simulink model "SistemaEstanques_PID_discreto"  (R2022a)
settings: Solver=ode3  StartTime=0.0  StopTime=3600*30  FixedStep=0.05  RelTol=1e-3  EnableMultiTasking=on
undefined symbols (not defined in the file or in its folder): gaussian, magnitude
libraries: simulink x5, slpidlib x1
settings Model: PauseTimes=10  PacingRate=100  Creator=Cristian  LastModifiedBy=Joaquín
settings SolverCC: AlgebraicLoopSolver=TrustRegion
settings DataIOCC: LimitDataPoints=on  SaveFormat=Array  ReturnWorkspaceOutputs=off
settings OptimizationCC: LifeSpan=inf
settings DebuggingCC: UnderspecifiedInitializationDetection=Classic  MergeDetectMultiDrivingBlocksExec=none  SolverPrmCheckMsg=warning  MultiTaskRateTransMsg=warning  UnconnectedInputMsg=warning  UnconnectedOutputMsg=warning  UnconnectedLineMsg=warning  StateNameClashWarn=warning  SFUnexpectedBacktrackingDiag=warning  SFNoUnconditionalDefaultTransitionDiag=warning  SFExecutionAtInitializationDiag=none  SFMachineParentedDataDiag=warning  ArithmeticOperatorsInVariantConditions=warning
settings HardwareCC: ProdBitPerPointer=32  ProdBitPerSizeT=32  ProdBitPerPtrDiffT=32  ProdLargestAtomicFloat=None  ProdIntDivRoundTo=Undefined  ProdEndianess=Unspecified  ProdWordSize=32  ProdHWDeviceType=32-bit Generic
settings ModelReferenceCC: PropagateSignalLabelsOutOfModel=off
settings SFSimCC: SimUseLocalCustomCode=off  CustomCodeUndefinedFunction=UseInterfaceOnly
settings RTWCC: RTWUseLocalCustomCode=off
settings CodeAppCC: StateflowObjectComments=on
settings GRTTargetCC: TargetLangStandard=C89/C90 (ANSI)
settings ConfigComp: CovMetricSettings=dw  CovSaveCumulativeToWorkspaceVar=on  CovSaveSingleToWorkspaceVar=on  CovExternalEMLEnable=off

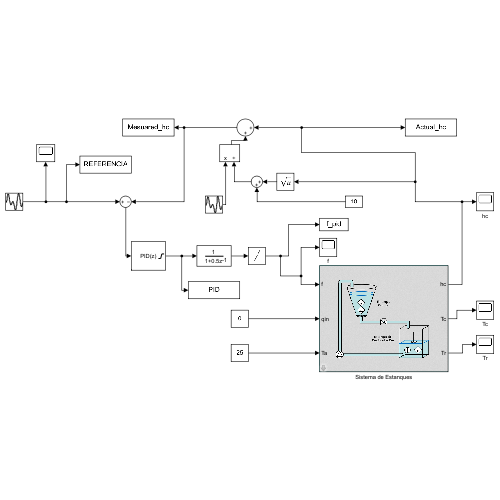
[thumbnail: Simulink's stored preview of the top-level diagram]
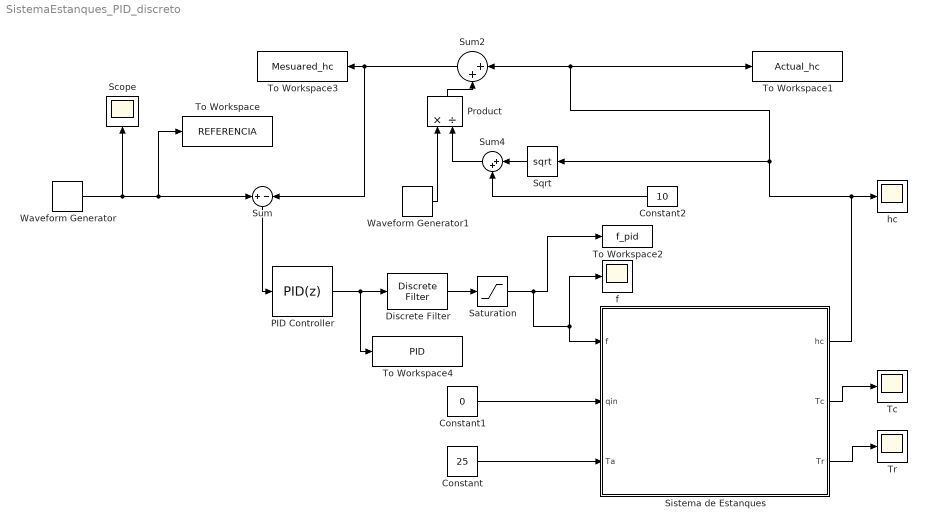
== system SistemaEstanques_PID_discreto ==
  Constant : Constant  Value=25
  Constant1 : Constant  Value=0
  Constant2 : Constant  Value=10
  Discrete Filter : DiscreteFilter
  PID Controller : slpidlib/PID Controller  Controller=PID  Form=Parallel  TimeDomain=Discrete-time  UseExternalTs=off  SampleTime=30  IntegratorMethod=Forward Euler  FilterMethod=Forward Euler  ControllerParametersSource=internal  P=107.25/5  I=9.41*10^(-5)  UseKiTs=off  D=4.44  N=0  UseFilter=on  TunerSelectOption=Transfer Function Based (PID Tuner App)  ZeroCross=off  InitialConditionSource=internal  InitialConditionForIntegrator=0  InitialConditionForFilter=0.00000001  DifferentiatorICPrevScaledInput=0  ExternalReset=none  IgnoreLimit=on  TrackingMode=off  Kt=1  LimitOutput=on  SatLimitsSource=internal  UpperSaturationLimit=100  LowerSaturationLimit=0  LinearizeAsGain=on  AntiWindupMode=none  Kb=1  RndMeth=Nearest  POutMin=[]  POutMax=[]  IOutMin=[]  IOutMax=[]  DOutMin=[]  DOutMax=[]  NOutMin=[]  NOutMax=[]  SumOutMin=[]  SumOutMax=[]  SaturationOutMin=[]  SaturationOutMax=[]  PParamMin=[]  PParamMax=[]  IParamMin=[]  IParamMax=[]  DParamMin=[]  DParamMax=[]  NParamMin=[]  NParamMax=[]  KbParamMin=[]  KbParamMax=[]  KtParamMin=[]  KtParamMax=[]  KbOutMin=[]  KbOutMax=[]  KtOutMin=[]  KtOutMax=[]  IntegratorOutMin=[]  IntegratorOutMax=[]  FilterOutMin=[]  FilterOutMax=[]  SumI1OutMin=[]  SumI1OutMax=[]  SumI2OutMin=[]  SumI2OutMax=[]  SumI3OutMin=[]  SumI3OutMax=[]  SumI4OutMin=[]  SumI4OutMax=[]  SumDOutMin=[]  SumDOutMax=[]  DifferentiatorOutMin=[]  DifferentiatorOutMax=[]  FilterDiffOutCoefMin=[]  FilterDiffOutCoefMax=[]  ReciprocalOutMin=[]  ReciprocalOutMax=[]  SumDenOutMin=[]  SumDenOutMax=[]  SumNumOutMin=[]  SumNumOutMax=[]  DivideOutMin=[]  DivideOutMax=[]  UdiffTsProdOutMin=[]  UdiffTsProdOutMax=[]  NTsProdOutMin=[]  NTsProdOutMax=[]  UintegralTsProdOutMin=[]  UintegralTsProdOutMax=[]  UngainTsProdOutMin=[]  UngainTsProdOutMax=[]  IntegratorContinuousStateAttributes=''  IntegratorStateMustResolveToSignalObject=off  IntegratorRTWStateStorageClass=Auto  FilterContinuousStateAttributes=''  FilterStateMustResolveToSignalObject=off  FilterRTWStateStorageClass=Auto  ParallelPVariant=InternalParameters  IdealPVariant=Disabled  IVariant=InternalParameters  DVariant=InternalParameters  IntegratorVariant=Discrete  SatVariant=Enabled  AWVariant=Passthrough  PCopyVariant=Disabled  TRVariant=Disabled  FdbkBlocksVariant=Forward  IdealPFdbkVariant=Disabled  SatFdbkVariant=Disabled  DerivativeFilterVariant=ForwardEulerFilter  NVariant=InternalParameters  NCopyVariant=Disabled  FilterICVariant=InternalICsFilter  IntegratorICVariant=InternalICs  ExternalResetVariant=Disabled  TRSumVariant=Passthrough  SumFdbkVariant=Disabled  SumVariant=Sum_PID  TsampFilterVariant=InternalTs  TsampNgainVariant=Passthrough  TsampIntegralVariant=Passthrough  ExternalSaturationOutDataTypeStr=Inherit: Same as second input  aMode=0
      settings: LockScale=on
  Product : Product  Inputs=*/
  Saturation : Saturate  UpperLimit=99.99  LowerLimit=0.01
  Scope : Scope
  Sistema de Estanques : Subsystem  mask(Sistema de Estanques){h0=0, T0c=15, T0r=15, Fout_null=off}
      mask prompts: h0 "Nivel inicial estanque cónico [cm]"; T0c "Temperatura inicial cónico [°C]"; T0r "Temperatura inicial recirculación [°C]"; Fout_null "Flujo de salida nulo"
      mask help:
      | Modelo de Sistema de Estanques del Laboratorio de Automática, Departamento de Ingeniería Eléctrica, Universidad de Chile.
      |
      | Desarrollado por: C. Jáuregui.
      | cjauregui@ing.uchile.cl
      mask init:
      | % Flujos entrada/salida
      | alpha1 = 5.4315;    %[cm3/s%]
      | alpha2 = -78.2333;  %[cm3/s]
      | beta = 20.21;       %[cm5/2/s]
      | 
      | % Dimensiones estanques
      | d = 50;    %[cm]
      | R = 34.5;  %[cm]
      | H = 79.8;  %[cm]
      | e = 0.3;   %[cm)
      | 
      | % Propiedades líquido
      | rho = 1;       %[g/cm3]
      | cp = 4.186;    %[J/g°C]
      | M = 137500;    %[g]
      | 
      | % Coeficientes
      | ha = 0.0054035;        %[J/s cm2 °C]
      | km = 2.7087*10^(-12);  %[J/s cm °C]
      mask Display:
      | image('SistemaEstanques.png')
      | 
      | port_label('input',1,'f')
      | port_label('input',2,'qin')
      | port_label('input',3,'Ta')
      | 
      | 
      | port_label('output',1,'hc')
      | port_label('output',2,'Tc')
      | port_label('output',3,'Tr')
  Sqrt : Sqrt
  Sum : Sum  Inputs=+|-
  Sum2 : Sum  Inputs=|++
  Sum4 : Sum  Inputs=|++
  Tc : Scope
  To Workspace : ToWorkspace  VariableName=REFERENCIA  SaveFormat=Timeseries  SampleTime=1
  To Workspace1 : ToWorkspace  VariableName=Actual_hc  SaveFormat=Timeseries  SampleTime=1
  To Workspace2 : ToWorkspace  VariableName=f_pid  SaveFormat=Timeseries  SampleTime=1
  To Workspace3 : ToWorkspace  VariableName=Mesuared_hc  SaveFormat=Timeseries  SampleTime=1
  To Workspace4 : ToWorkspace  VariableName=PID  SaveFormat=Timeseries  SampleTime=-1
  Tr : Scope
  Waveform Generator : simulink/Sources/Waveform Generator  OutMin=[]  OutMax=[]  OutDataTypeStr=double  SelectedSignal=1  Signals=step(0,0,40)+step(400,0,-25)+step(800,0,16)+step(1200,0,14)+step(1600,0,3)+step(2000,0,-10)+step(2400,0,-18)+step(2800,0,6)+step(3200,0,-1)+step(3600,0,19)+step(4000,0,-2)+step(4400,0,-39)+step(4800,0,13)+step(5200,0,1)+step(5600,0,33)+step(6000,0,-42)+step(6400,0,33)+step(6800,0,-5)+step(7200,0,5)+step(7600,0,-38)+step(8000,0,34)+step(8400,0,-11)+step(8800,0,-6)+step(9200,0,8)+step(9600,0,11)+step(10000,0,-20)+step(10400,0,8)+step(10800,0,11)+step(11200,0,-38)+step(11600,0,33)+step(12000,0,12)+step(12400,0,-35)+step(12800,0,39)+step(13200,0,-23)+step(13600,0,13)+step(14000,0,0)+step(14400,0,-11)+step(14800,0,13)+step(15200,0,-12)+step(15600,0,18)+step(16000,0,-16)+step(16400,0,-29)+step(16800,0,17)+step(17200,0,-5)+step(17600,0,2)+step(18000,0,0)+step(18400,0,-16)+step(18800,0,50)+step(19200,0,-24)+step(19600,0,-11)+step(20000,0,24)+step(20400,0,-14)+step(20800,0,9)+step(21200,0,-30)+step(21600,0,34)+step(22000,0,-6)+step(22400,0,16)+step(22800,0,-10)+step(23200,0,-34)+step(23600,0,29)+step(24000,0,4)+step(24400,0,-31)+step(24800,0,-2)+step(25200,0,33)+step(25600,0,9)+step(26000,0,-44)+step(26400,0,1)+step(26800,0,23)+step(27200,0,8)+step(27600,0,2)+step(28000,0,3)+step(28400,0,-28)+step(28800,0,32)+step(29200,0,6)+step(29600,0,1)+step(30000,0,-47)+step(30400,0,18)+step(30800,0,27)+step(31200,0,-34)+step(31600,0,29)+step(32000,0,-1)+step(32400,0,-23)+step(32800,0,31)+step(33200,0,-26)+step(33600,0,-23)+step(34000,0,35)+step(34400,0,-14)+step(34800,0,2)+step(35200,0,10)+step(35600,0,-18)+step(36000,0,10)+step(36400,0,-12)+step(36800,0,36)+step(37200,0,0)+step(37600,0,-29)+step(38000,0,9)+step(38400,0,18)+step(38800,0,-31)+step(39200,0,6)+step(39600,0,4)+step(40000,0,15)+step(40400,0,-36)+step(40800,0,38)+step(41200,0,-32)+step(41600,0,38)+step(42000,0,-3)+step(42400,0,-41)+step(42800,0,29)+step(43200,0,15)+step(43600,0,-10)+step(44000,0,8)+step(44400,0,-25)+step(44800,0,-9)+step(45200,0,-2)+step(45600,0,28)+step(46000,0,-39)+step(46400,0,29)+step(46800,0,6)+step(47200,0,9)+step(47600,0,2)+step(48000,0,-44)+step(48400,0,36)+step(48800,0,-30)+step(49200,0,18)+step(49600,0,-22)+step(50000,0,30)+step(50400,0,-16)+step(50800,0,26)+step(51200,0,-5)+step(51600,0,0)+step(52000,0,-3)+step(52400,0,-4)+step(52800,0,0)+step(53200,0,-32)+step(53600,0,4)+step(54000,0,5)+step(54400,0,14)+step(54800,0,-20)+step(55200,0,5)+step(55600,0,3)+step(56000,0,25)+step(56400,0,-11)+step(56800,0,24)+step(57200,0,-49)+step(57600,0,32)+step(58000,0,-25)+step(58400,0,38)+step(58800,0,-39)+step(59200,0,3)+step(59600,0,4)+step(60000,0,-13)+step(60400,0,31)+step(60800,0,-8)+step(61200,0,0)+step(61600,0,-22)+step(62000,0,16)+step(62400,0,19)+step(62800,0,-32)+step(63200,0,-1)+step(63600,0,-4)+step(64000,0,23)+step(64400,0,-22)+step(64800,0,45)+step(65200,0,-18)+step(65600,0,-1)+step(66000,0,-24)+step(66400,0,22)+step(66800,0,-18)+step(67200,0,0)+step(67600,0,-1)+step(68000,0,42)+step(68400,0,-37)+step(68800,0,-9)+step(69200,0,-1)+step(69600,0,4)+step(70000,0,12)+step(70400,0,33)+step(70800,0,-46)+step(71200,0,14)+step(71600,0,18)+step(72000,0,-36)+step(72400,0,5)+step(72800,0,26)+step(73200,0,-24)+step(73600,0,21)+step(74000,0,0)+step(74400,0,17)+step(74800,0,-24)+step(75200,0,-13)+step(75600,0,29)+step(76000,0,11)+step(76400,0,-18)+step(76800,0,19)+step(77200,0,-17)+step(77600,0,-13)+step(78000,0,-9)+step(78400,0,-3)+step(78800,0,22)+step(79200,0,4)+step(79600,0,-6)+step(80000,0,12)+step(80400,0,-33)+step(80800,0,34)+step(81200,0,-13)+step(81600,0,8)+step(82000,0,-21)+step(82400,0,20)+step(82800,0,-8)+step(83200,0,15)+step(83600,0,-23)+step(84000,0,18)+step(84400,0,-5)+step(84800,0,-24)+step(85200,0,-2)+step(85600,0,6)+step(86000,0,20)+step(86400,0,-6)+step(86800,0,-14)+step(87200,0,6)+step(87600,0,20)+step(88000,0,-29)+step(88400,0,-5)+step(88800,0,35)+step(89200,0,-26)+step(89600,0,6)+step(90000,0,7)+step(90400,0,-18)+step(90800,0,21)+step(91200,0,10)+step(91600,0,6)+step(92000,0,-26)+step(92400,0,14)+step(92800,0,2)+step(93200,0,-19)+step(93600,0,16)+step(94000,0,3)+step(94400,0,-2)+step(94800,0,-15)+step(95200,0,12)+step(95600,0,14)+step(96000,0,-31)+step(96400,0,29)+step(96800,0,-9)+step(97200,0,11)+step(97600,0,-34)+step(98000,0,11)+step(98400,0,2)+step(98800,0,-14)+step(99200,0,-1)+step(99600,0,11)+step(100000,0,29)+step(100400,0,-38)+step(100800,0,29)+step(101200,0,-14)+step(101600,0,12)+step(102000,0,3)+step(102400,0,-9)+step(102800,0,-5)+step(103200,0,5)+step(103600,0,17)+step(104000,0,-25)+step(104400,0,-17)+step(104800,0,8)+step(105200,0,22)+step(105600,0,12)+step(106000,0,-17)+step(106400,0,-17)+step(106800,0,22)+step(107200,0,-18)+step(107600,0,6)+step(108000,0,-13)+step(108400,0,40)+step(108800,0,0)+step(109200,0,-17)+step(109600,0,-8)+step(110000,0,5)+step(110400,0,-4)+step(110800,0,-16)+step(111200,0,14)+step(111600,0,25)+step(112000,0,-20)+step(112400,0,-7)+step(112800,0,-12)+step(113200,0,42)+step(113600,0,-34)+step(114000,0,38)+step(114400,0,-2)+step(114800,0,-14)+step(115200,0,10)+step(115600,0,40)+step(116000,0,-33)+step(116400,0,38)+step(116800,0,-16)+step(117200,0,-9)+step(117600,0,28)+step(118000,0,-31)+step(118400,0,3)+step(118800,0,7)+step(119200,0,18)+step(119600,0,-13)+step(120000,0,6)+step(120400,0,-2)+step(120800,0,-20)+step(121200,0,0)+step(121600,0,7)+step(122000,0,-3)+step(122400,0,-18)+step(122800,0,-2)+step(123200,0,21)+step(123600,0,12)+step(124000,0,-22)+step(124400,0,-4)+step(124800,0,37)+step(125200,0,-11)+step(125600,0,-20)+step(126000,0,-2)+step(126400,0,20)+step(126800,0,-31)+step(127200,0,43)+step(127600,0,-35)+step(128000,0,-4)+step(128400,0,37)+step(128800,0,-18)+step(129200,0,-14)+step(129600,0,5)+step(130000,0,25)+step(130400,0,-7)+step(130800,0,-28)+step(131200,0,45)+step(131600,0,-16)+step(132000,0,-1)+step(132400,0,-12)+step(132800,0,-8)+step(133200,0,-9)+step(133600,0,36)+step(134000,0,-21)+step(134400,0,27)+step(134800,0,-26)+step(135200,0,11)+step(135600,0,15)+step(136000,0,-31)+step(136400,0,30)+step(136800,0,-5)+step(137200,0,-17)+step(137600,0,-19)+step(138000,0,38)+step(138400,0,-7)+step(138800,0,15)+step(139200,0,-47)+step(139600,0,41)+step(140000,0,-16)+step(140400,0,0)+step(140800,0,8)+step(141200,0,11)+step(141600,0,-46)+step(142000,0,17)+step(142400,0,-12)+step(142800,0,0)+step(143200,0,25)+step(143600,0,-1)+step(144000,0,14)+step(144400,0,-32)+step(144800,0,29)+step(145200,0,1)+step(145600,0,-1)+step(146000,0,-19)+step(146400,0,-9)+step(146800,0,8)+step(147200,0,4)+step(147600,0,3)+step(148000,0,-17)+step(148400,0,2)+step(148800,0,-6)+step(149200,0,-1)+step(149600,0,29)+step(150000,0,9)+step(150400,0,4)+step(150800,0,-45)+step(151200,0,46)+step(151600,0,-3)+step(152000,0,-22)+step(152400,0,-17)+step(152800,0,36)+step(153200,0,-42)+step(153600,0,20)+step(154000,0,14)+step(154400,0,-33)+step(154800,0,38)+step(155200,0,-28)+step(155600,0,-4)+step(156000,0,-4)+step(156400,0,24)+step(156800,0,12)+step(157200,0,-31)+step(157600,0,-1)+step(158000,0,14)+step(158400,0,10)+step(158800,0,3)+step(159200,0,6)+step(159600,0,-23)+step(160000,0,22)+step(160400,0,-4)+step(160800,0,-15)+step(161200,0,26)+step(161600,0,-34)+step(162000,0,28)+step(162400,0,-33)+step(162800,0,40)+step(163200,0,-8)+step(163600,0,-2)+step(164000,0,-30)+step(164400,0,40)+step(164800,0,-41)+step(165200,0,26)+step(165600,0,-8)+step(166000,0,20)+step(166400,0,-27)+step(166800,0,-4)+step(167200,0,36)+step(167600,0,-10)+step(168000,0,-36)+step(168400,0,5)+step(168800,0,26)+step(169200,0,-9)+step(169600,0,-3)+step(170000,0,21)+step(170400,0,-2)+step(170800,0,-3)+step(171200,0,-17)+step(171600,0,-19)+step(172000,0,8)+step(172400,0,14)+step(172800,0,-3)+step(173200,0,9)+step(173600,0,-20)+step(174000,0,-3)+step(174400,0,11)+step(174800,0,22)+step(175200,0,0)+step(175600,0,1)+step(176000,0,-14)+step(176400,0,15)+step(176800,0,-36)+step(177200,0,32)+step(177600,0,-17)+step(178000,0,3)+step(178400,0,-17)+step(178800,0,37)+step(179200,0,-35)+step(179600,0,13)+step(180000,0,-22)+step(180400,0,0)+step(180800,0,9)+step(181200,0,13)+step(181600,0,-1)+step(182000,0,-13)+step(182400,0,-5)+step(182800,0,-2)+step(183200,0,15)+step(183600,0,20)+step(184000,0,-35)+step(184400,0,10)+step(184800,0,25)+step(185200,0,-31)+step(185600,0,24)+step(186000,0,-16)+step(186400,0,22)+step(186800,0,-3)+step(187200,0,-27)+step(187600,0,10)+step(188000,0,-11)+step(188400,0,28)+step(188800,0,13)+step(189200,0,-29)+step(189600,0,8)+step(190000,0,-10)+step(190400,0,-6)+step(190800,0,-7)+step(191200,0,46)+step(191600,0,-26)+step(192000,0,7)+step(192400,0,17)+step(192800,0,-43)+step(193200,0,14)+step(193600,0,7)+step(194000,0,-10)+step(194400,0,-12)+step(194800,0,17)+step(195200,0,15)+step(195600,0,-24)+step(196000,0,-4)+step(196400,0,3)+step(196800,0,-2)+step(197200,0,35)+step(197600,0,-8)+step(198000,0,4)+step(198400,0,-15)+step(198800,0,15)+step(199200,0,-32)+step(199600,0,11)+step(200000,0,12)+step(200400,0,0)+step(200800,0,20)+step(201200,0,-38)+step(201600,0,5)+step(202000,0,-8)+step(202400,0,41)+step(202800,0,-5)+step(203200,0,-8)+step(203600,0,0)+step(204000,0,-6)+step(204400,0,-8)+step(204800,0,-5)+step(205200,0,10)+step(205600,0,-14)+step(206000,0,27)+step(206400,0,-22)+step(206800,0,9)+step(207200,0,-22)+step(207600,0,2)+step(208000,0,41)+step(208400,0,-18)+step(208800,0,-22)+step(209200,0,-7)+step(209600,0,16)+step(210000,0,-7)+step(210400,0,34)+step(210800,0,-14)+step(211200,0,9)+step(211600,0,-18)+step(212000,0,16)+step(212400,0,8)+step(212800,0,-24)+step(213200,0,-7)+step(213600,0,11)+step(214000,0,0)+step(214400,0,-16)+step(214800,0,39)+step(215200,0,2)+step(215600,0,-45)+step(216000,0,40)+step(216400,0,-4)+step(216800,0,-6)+step(217200,0,-2)+step(217600,0,13)+step(218000,0,-36)+step(218400,0,15)+step(218800,0,12)+step(219200,0,-4)+step(219600,0,-15)+step(220000,0,8)+step(220400,0,-10)+step(220800,0,39)+step(221200,0,-8)+step(221600,0,-5)+step(222000,0,12)+step(222400,0,1)+step(222800,0,-49)+step(223200,0,43)+step(223600,0,5)+step(224000,0,40)+step(224400,0,-14)+step(224800,0,1)+step(225200,0,-12)+step(225600,0,-5)+step(226000,0,5)+step(226400,0,4)+step(226800,0,3)+step(227200,0,-9)+step(227600,0,2)+step(228000,0,20)+step(228400,0,-19)+step(228800,0,25)+step(229200,0,-12)+step(229600,0,13)+step(230000,0,-40)+step(230400,0,0)+step(230800,0,2)+step(231200,0,40)+step(231600,0,-25)+step(232000,0,18)+step(232400,0,8)+step(232800,0,-13)+step(233200,0,-16)+step(233600,0,4)+step(234000,0,7)+step(234400,0,-10)+step(234800,0,16)+step(235200,0,-24)+step(235600,0,31)+step(236000,0,-11)+step(236400,0,-3)+step(236800,0,-11)+step(237200,0,26)+step(237600,0,-1)+step(238000,0,7)+step(238400,0,-38)+step(238800,0,1)+step(239200,0,0)+step(239600,0,30)+step(240000,0,-3)+step(240400,0,-26)+step(240800,0,0)+step(241200,0,30)+step(241600,0,-26)+step(242000,0,31)+step(242400,0,0)+step(242800,0,1)+step(243200,0,-25)+step(243600,0,19)+step(244000,0,-15)+step(244400,0,8)+step(244800,0,13)+step(245200,0,-7)+step(245600,0,-16)+step(246000,0,7)+step(246400,0,11)+step(246800,0,-30)+step(247200,0,-3)+step(247600,0,13)+step(248000,0,7)+step(248400,0,-22)+step(248800,0,46)+step(249200,0,-34)+step(249600,0,1)+step(250000,0,8)+step(250400,0,-16)+step(250800,0,18)+step(251200,0,20)+step(251600,0,-1)+step(252000,0,-34)+step(252400,0,-1)+step(252800,0,-8)+step(253200,0,36)+step(253600,0,-15)+step(254000,0,-3)+step(254400,0,22)+step(254800,0,-10)+step(255200,0,-4)+step(255600,0,-14)+step(256000,0,29)+step(256400,0,-7)+step(256800,0,3)+step(257200,0,-16)+step(257600,0,4)+step(258000,0,17)+step(258400,0,-17)+step(258800,0,3)+step(259200,0,-13)+step(259600,0,-16)+step(260000,0,10)+step(260400,0,24)+step(260800,0,-7)+step(261200,0,-6)+step(261600,0,13)+step(262000,0,-19)+step(262400,0,26)+step(262800,0,-26)+step(263200,0,6)+step(263600,0,11)+step(264000,0,-19)+step(264400,0,-3)+step(264800,0,35)+step(265200,0,-2)+step(265600,0,-15)+step(266000,0,-5)+step(266400,0,7)+step(266800,0,-18)+step(267200,0,9)+step(267600,0,5)+step(268000,0,-4)+step(268400,0,6)+step(268800,0,18)+step(269200,0,-14)+step(269600,0,-14)+step(270000,0,7)+step(270400,0,-7)+step(270800,0,-3)+step(271200,0,18)+step(271600,0,2)+step(272000,0,-11)+step(272400,0,-4)+step(272800,0,5)+step(273200,0,-20)+step(273600,0,-4)+step(274000,0,13)+step(274400,0,-9)+step(274800,0,1)+step(275200,0,1)+step(275600,0,9)+step(276000,0,17)+step(276400,0,-8)+step(276800,0,-4)+step(277200,0,19)+step(277600,0,1)+step(278000,0,8)+step(278400,0,-19)+step(278800,0,-1)+step(279200,0,3)+step(279600,0,16)+step(280000,0,-45)+step(280400,0,16)+step(280800,0,28)+step(281200,0,-48)+step(281600,0,34)+step(282000,0,-31)+step(282400,0,26)+step(282800,0,4)+step(283200,0,15)+step(283600,0,2)+step(284000,0,-44)+step(284400,0,26)+step(284800,0,-30)+step(285200,0,14)+step(285600,0,18)+step(286000,0,14)+step(286400,0,2)+step(286800,0,-17)+step(287200,0,-26)+step(287600,0,6)+step(288000,0,18)+step(288400,0,14)+step(288800,0,-13)+step(289200,0,-25)+step(289600,0,20)+step(290000,0,-1)+step(290400,0,1)+step(290800,0,-8)+step(291200,0,18)+step(291600,0,4)+step(292000,0,-27)+step(292400,0,18)+step(292800,0,16)+step(293200,0,-18)+step(293600,0,-20)+step(294000,0,-3)+step(294400,0,30)+step(294800,0,-21)+step(295200,0,18)+step(295600,0,5)+step(296000,0,4)+step(296400,0,-5)+step(296800,0,-14)+step(297200,0,-11)+step(297600,0,30)+step(298000,0,-29)+step(298400,0,27)+step(298800,0,-35)+step(299200,0,15)+step(299600,0,24)+step(300000,0,-42)+step(300400,0,18)+step(300800,0,14)+step(301200,0,5)+step(301600,0,-22)+step(302000,0,-4)+step(302400,0,35)+step(302800,0,-43)+step(303200,0,18)+step(303600,0,3)+step(304000,0,-14)+step(304400,0,18)+step(304800,0,-23)+step(305200,0,19)+step(305600,0,-18)+step(306000,0,36)+step(306400,0,-9)+step(306800,0,12)+step(307200,0,-25)+step(307600,0,2)+step(308000,0,11)+step(308400,0,-31)+step(308800,0,22)+step(309200,0,8)+step(309600,0,9)+step(310000,0,3)+step(310400,0,-15)+step(310800,0,-3)+step(311200,0,-22)+step(311600,0,30)+step(312000,0,-37)+step(312400,0,50)+step(312800,0,-40)+step(313200,0,-7)+step(313600,0,4)+step(314000,0,42)+step(314400,0,-10)+step(314800,0,6)+step(315200,0,2)+step(315600,0,-17)+step(316000,0,-29)+step(316400,0,20)+step(316800,0,23)+step(317200,0,-28)+step(317600,0,-9)+step(318000,0,-7)+step(318400,0,11)+step(318800,0,-2)+step(319200,0,-8)+step(319600,0,41)+step(320000,0,-17)+step(320400,0,16)+step(320800,0,-9)+step(321200,0,-12)+step(321600,0,1)+step(322000,0,11)+step(322400,0,-9)+step(322800,0,12)+step(323200,0,-8)+step(323600,0,7)+step(324000,0,0)+step(324400,0,-27)+step(324800,0,38)+step(325200,0,-42)+step(325600,0,20)+step(326000,0,17)+step(326400,0,8)+step(326800,0,-37)+step(327200,0,18)+step(327600,0,13)+step(328000,0,-21)+step(328400,0,-17)+step(328800,0,26)+step(329200,0,0)+step(329600,0,5)+step(330000,0,14)+step(330400,0,-20)+step(330800,0,-24)+step(331200,0,44)+step(331600,0,40)+step(332000,0,-16)+step(332400,0,-17)+step(332800,0,35)+step(333200,0,-1)+step(333600,0,-36)+step(334000,0,11)+step(334400,0,-11)+step(334800,0,45)+step(335200,0,-4)+step(335600,0,-32)+step(336000,0,33)+step(336400,0,-38)+step(336800,0,34)+step(337200,0,-12)+step(337600,0,15)+step(338000,0,-12)+step(338400,0,-16)+step(338800,0,7)+step(339200,0,-19)+step(339600,0,40)+step(340000,0,-10)+step(340400,0,13)+step(340800,0,-21)+step(341200,0,11)+step(341600,0,-12)+step(342000,0,-13)+step(342400,0,7)+step(342800,0,8)+step(343200,0,-20)+step(343600,0,24)+step(344000,0,13)+step(344400,0,-10)+step(344800,0,8)+step(345200,0,9)+step(345600,0,-6)+step(346000,0,-28)+step(346400,0,22)+step(346800,0,40)+step(347200,0,-18)+step(347600,0,8)+step(348000,0,-16)+step(348400,0,-14)+step(348800,0,29)+step(349200,0,-20)+step(349600,0,17)+step(350000,0,22)+step(350400,0,-38)+step(350800,0,4)+step(351200,0,-1)+step(351600,0,1)+step(352000,0,21)+step(352400,0,-35)+step(352800,0,44)+step(353200,0,1)+step(353600,0,-31)+step(354000,0,16)+step(354400,0,4)+step(354800,0,3)+step(355200,0,-35)+step(355600,0,41)+step(356000,0,-11)+step(356400,0,-11)+step(356800,0,-1)+step(357200,0,27)+step(357600,0,-3)+step(358000,0,-12)+step(358400,0,-17)+step(358800,0,2)+step(359200,0,9)+step(359600,0,18)+step(360000,0,-38)+step(360400,0,12)+step(360800,0,10)+step(361200,0,-12)+step(361600,0,-16)+step(362000,0,12)+step(362400,0,-7)+step(362800,0,37)+step(363200,0,3)+step(363600,0,-20)+step(364000,0,-9)+step(364400,0,-9)+step(364800,0,25)+step(365200,0,-24)+step(365600,0,7)+step(366000,0,17)+step(366400,0,-15)+step(366800,0,27)+step(367200,0,-23)+step(367600,0,-12)+step(368000,0,-6)+step(368400,0,13)+step(368800,0,18)+step(369200,0,-5)+step(369600,0,-28)+step(370000,0,46)+step(370400,0,-18)+step(370800,0,-1)+step(371200,0,19)+step(371600,0,-1)+step(372000,0,-1)+step(372400,0,-14)+step(372800,0,-4)+step(373200,0,15)+step(373600,0,-28)+step(374000,0,28)+step(374400,0,-8)+step(374800,0,1)+step(375200,0,-26)+step(375600,0,-8)+step(376000,0,7)+step(376400,0,0)+step(376800,0,24)+step(377200,0,-29)+step(377600,0,21)+step(378000,0,-4)+step(378400,0,-20)+step(378800,0,15)+step(379200,0,9)+step(379600,0,-21)+step(380000,0,47)+step(380400,0,-12)+step(380800,0,10)+step(381200,0,-35)+step(381600,0,15)+step(382000,0,-20)+step(382400,0,17)+step(382800,0,16)+step(383200,0,-27)+step(383600,0,14)+step(384000,0,-16)+step(384400,0,16)+step(384800,0,11)+step(385200,0,-14)+step(385600,0,19)+step(386000,0,-21)+step(386400,0,-2)+step(386800,0,4)+step(387200,0,-2)+step(387600,0,-13)+step(388000,0,27)+step(388400,0,-8)+step(388800,0,-10)+step(389200,0,13)+step(389600,0,10)+step(390000,0,-32)+step(390400,0,-2)+step(390800,0,19)+step(391200,0,-19)+step(391600,0,14)+step(392000,0,-19)+step(392400,0,33)+step(392800,0,8)+step(393200,0,-36)+step(393600,0,5)+step(394000,0,1)+step(394400,0,22)+step(394800,0,-7)+step(395200,0,-11)+step(395600,0,7)+step(396000,0,-5)+step(396400,0,-11)  BlockNames=MultiportSwitch_8b811f9eeedb459  SampleTime=0.1
  Waveform Generator1 : simulink/Sources/Waveform Generator  OutMin=[]  OutMax=[]  OutDataTypeStr=double  SelectedSignal=1  Signals=gaussian(0,1,1)  BlockNames=MultiportSwitch_81c2e3fb5dc44a9  SampleTime=0.1
  f : Scope
  hc : Scope
  wires:
  Constant/1 -> Sistema de Estanques/3(Ta)
  Constant1/1 -> Sistema de Estanques/2(qin)
  Sistema de Estanques/3(Tr) -> Tr/1
  Sistema de Estanques/2(Tc) -> Tc/1
  Waveform Generator/1 -> Sum/1, To Workspace/1, Scope/1
  Sum2/1 -> Sum/2, To Workspace3/1
  Waveform Generator1/1 -> Product/1
  Product/1 -> Sum2/2
  Sistema de Estanques/1(hc) -> Sqrt/1, Sum2/1, To Workspace1/1, hc/1
  Constant2/1 -> Sum4/2
  Sum4/1 -> Product/2
  Sqrt/1 -> Sum4/1
  Sum/1 -> PID Controller/1
  Discrete Filter/1 -> Saturation/1
  Saturation/1 -> To Workspace2/1, f/1, Sistema de Estanques/1(f)
  PID Controller/1 -> To Workspace4/1, Discrete Filter/1

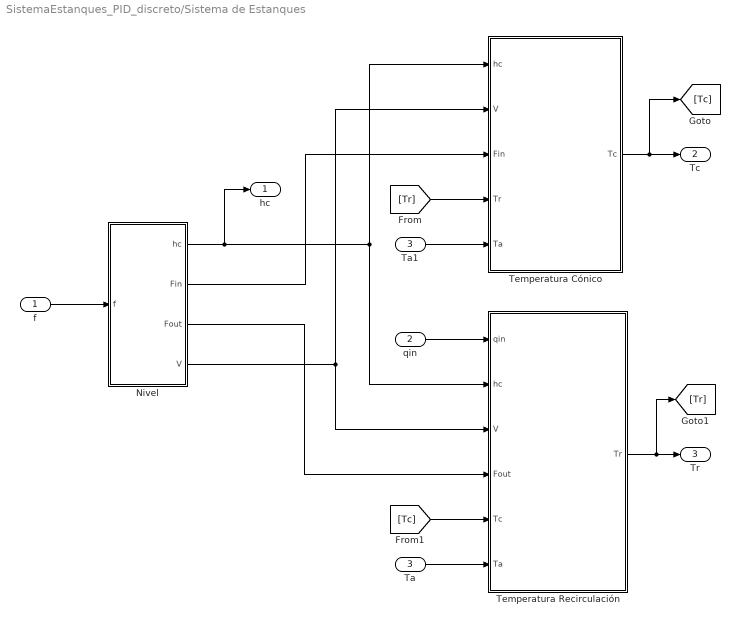
== system SistemaEstanques_PID_discreto/Sistema de Estanques ==
  f : Inport
  qin : Inport  Port=2
  Ta : Inport  Port=3
  Nivel : Subsystem
  Ta1 : InportShadow  Port=3
  Temperatura Cónico : Subsystem
  Temperatura Recirculación : Subsystem
  hc : Outport
  Tc : Outport  Port=2
  Tr : Outport  Port=3
  wires:
  f/1 -> Nivel/1(f)
  Temperatura Cónico/1(Tc) -> [Tc], Tc/1
  qin/1 -> Temperatura Recirculación/1(qin)
  Ta/1 -> Temperatura Recirculación/6(Ta)
  Nivel/1(hc) -> Temperatura Cónico/1(hc), Temperatura Recirculación/2(hc), hc/1
  Ta1/1 -> Temperatura Cónico/5(Ta)
  Nivel/4(V) -> Temperatura Cónico/2(V), Temperatura Recirculación/3(V)
  Nivel/2(Fin) -> Temperatura Cónico/3(Fin)
  Nivel/3(Fout) -> Temperatura Recirculación/4(Fout)
  Temperatura Recirculación/1(Tr) -> [Tr], Tr/1
  [Tr] -> Temperatura Cónico/4(Tr)
  [Tc] -> Temperatura Recirculación/5(Tc)

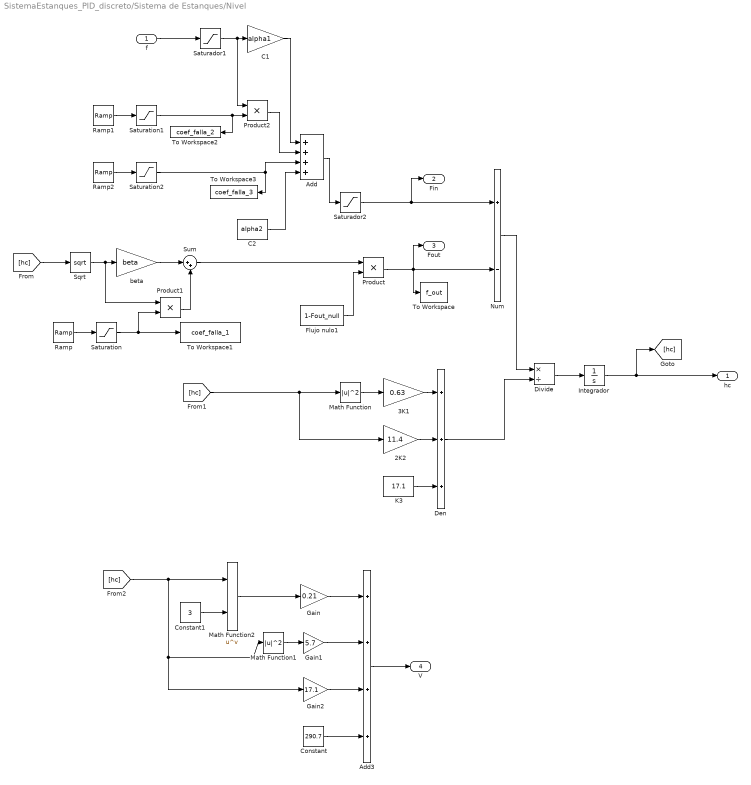
== system SistemaEstanques_PID_discreto/Sistema de Estanques/Nivel ==
  f : Inport
  2K2 : Gain  Gain=11.4
  3K1 : Gain  Gain=0.63
  Add : Sum  Inputs=++++
  Add3 : Sum  Inputs=++++
  C1 : Gain  Gain=alpha1
  C2 : Constant  Value=alpha2
  Constant : Constant  Value=290.7
  Constant1 : Constant  Value=3
  Den : Sum  Inputs=+++
  Divide : Product  Inputs=*/
  Flujo nulo1 : Constant  Value=1-Fout_null
  Gain : Gain  Gain=0.21
  Gain1 : Gain  Gain=5.7
  Gain2 : Gain  Gain=17.1
  Integrador : Integrator  InitialCondition=h0+10^(-6)  LimitOutput=on  LowerSaturationLimit=10^(-6)  ZeroCross=off
  K3 : Constant  Value=17.1
  Math Function : Math  Operator=magnitude^2  SignedPower=on
  Math Function1 : Math  Operator=magnitude^2  SignedPower=on
  Math Function2 : Math  Operator=pow  SignedPower=on
  Num : Sum  Inputs=+-
  Product : Product
  Product1 : Product
  Product2 : Product
  Ramp : simulink/Sources/Ramp  slope=0.0001  start=3600*10  InitialOutput=0
  Ramp1 : simulink/Sources/Ramp  slope=0.0001  start=3600*10  InitialOutput=0
  Ramp2 : simulink/Sources/Ramp  slope=0.0001  start=3600*10  InitialOutput=0
  Saturador1 : Saturate  UpperLimit=100  LowerLimit=0  ZeroCross=off
  Saturador2 : Saturate  UpperLimit=inf  LowerLimit=0  ZeroCross=off
  Saturation : Saturate  UpperLimit=0
  Saturation1 : Saturate  UpperLimit=200
  Saturation2 : Saturate  UpperLimit=0
  Sqrt : Sqrt
  Sum : Sum  Inputs=|++
  To Workspace : ToWorkspace  VariableName=f_out  SaveFormat=Timeseries  SampleTime=-1
  To Workspace1 : ToWorkspace  VariableName=coef_falla_1  SaveFormat=Timeseries  SampleTime=1
  To Workspace2 : ToWorkspace  VariableName=coef_falla_2  SaveFormat=Timeseries  SampleTime=-1
  To Workspace3 : ToWorkspace  VariableName=coef_falla_3  SaveFormat=Timeseries  SampleTime=-1
  beta : Gain  Gain=beta
  hc : Outport
  Fin : Outport  Port=2
  Fout : Outport  Port=3
  V : Outport  Port=4
  wires:
  [hc] -> Sqrt/1
  3K1/1 -> Den/1
  K3/1 -> Den/3
  [hc] -> 2K2/1, Math Function/1
  C2/1 -> Add/4
  C1/1 -> Add/1
  Num/1 -> Divide/1
  Divide/1 -> Integrador/1
  Math Function/1 -> 3K1/1
  2K2/1 -> Den/2
  Den/1 -> Divide/2
  Saturador2/1 -> Fin/1, Num/1
  Saturador1/1 -> Product2/1, C1/1
  Add/1 -> Saturador2/1
  f/1 -> Saturador1/1
  Integrador/1 -> hc/1, [hc]
  Constant/1 -> Add3/4
  Gain/1 -> Add3/1
  Gain1/1 -> Add3/2
  Gain2/1 -> Add3/3
  Math Function1/1 -> Gain1/1
  Constant1/1 -> Math Function2/2
  Math Function2/1 -> Gain/1
  [hc] -> Gain2/1, Math Function1/1, Math Function2/1
  Add3/1 -> V/1
  Product/1 -> To Workspace/1, Fout/1, Num/2
  Flujo nulo1/1 -> Product/2
  beta/1 -> Sum/1
  Ramp/1 -> Saturation/1
  Sum/1 -> Product/1
  Sqrt/1 -> Product1/1, beta/1
  Product1/1 -> Sum/2
  Saturation/1 -> To Workspace1/1, Product1/2
  Saturation1/1 -> To Workspace2/1, Product2/2
  Ramp1/1 -> Saturation1/1
  Product2/1 -> Add/2
  Ramp2/1 -> Saturation2/1
  Saturation2/1 -> To Workspace3/1, Add/3

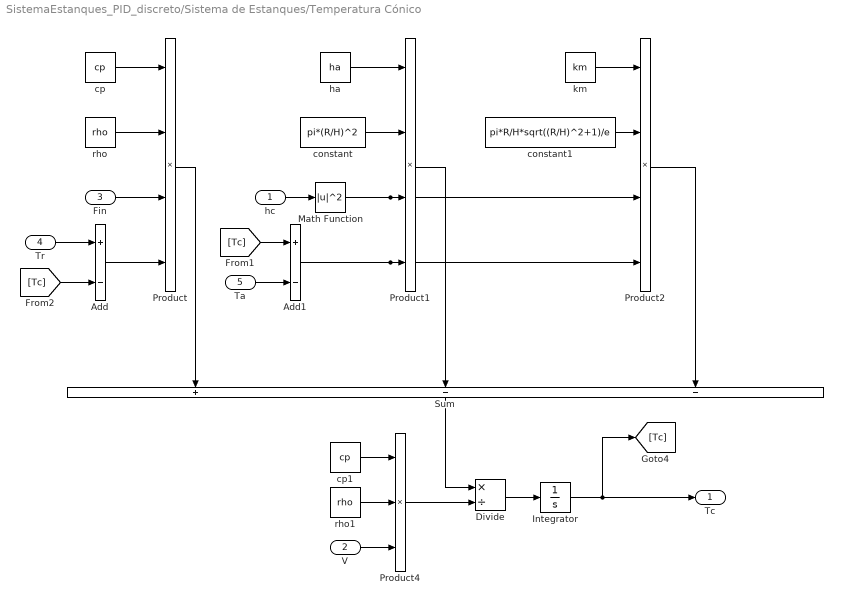
== system SistemaEstanques_PID_discreto/Sistema de Estanques/Temperatura Cónico ==
  hc : Inport
  V : Inport  Port=2
  Fin : Inport  Port=3
  Tr : Inport  Port=4
  Ta : Inport  Port=5
  Add : Sum  Inputs=+-
  Add1 : Sum  Inputs=+-
  Divide : Product  Inputs=*/
  Integrator : Integrator  InitialCondition=T0c
  Math Function : Math  Operator=magnitude^2  SignedPower=on
  Product : Product  Inputs=4
  Product1 : Product  Inputs=4
  Product2 : Product  Inputs=4
  Product4 : Product  Inputs=3
  Sum : Sum  Inputs=+--
  constant : Constant  Value=pi*(R/H)^2
  constant1 : Constant  Value=pi*R/H*sqrt((R/H)^2+1)/e
  cp : Constant  Value=cp
  cp1 : Constant  Value=cp
  ha : Constant  Value=ha
  km : Constant  Value=km
  rho : Constant  Value=rho
  rho1 : Constant  Value=rho
  Tc : Outport
  wires:
  Integrator/1 -> Tc/1, [Tc]
  cp/1 -> Product/1
  rho/1 -> Product/2
  Fin/1 -> Product/3
  Add/1 -> Product/4
  hc/1 -> Math Function/1
  [Tc] -> Add/2
  Tr/1 -> Add/1
  [Tc] -> Add1/1
  Ta/1 -> Add1/2
  ha/1 -> Product1/1
  constant/1 -> Product1/2
  Math Function/1 -> Product2/3, Product1/3
  Add1/1 -> Product1/4, Product2/4
  km/1 -> Product2/1
  constant1/1 -> Product2/2
  Product/1 -> Sum/1
  Product1/1 -> Sum/2
  Product2/1 -> Sum/3
  Product4/1 -> Divide/2
  Sum/1 -> Divide/1
  Divide/1 -> Integrator/1
  cp1/1 -> Product4/1
  rho1/1 -> Product4/2
  V/1 -> Product4/3

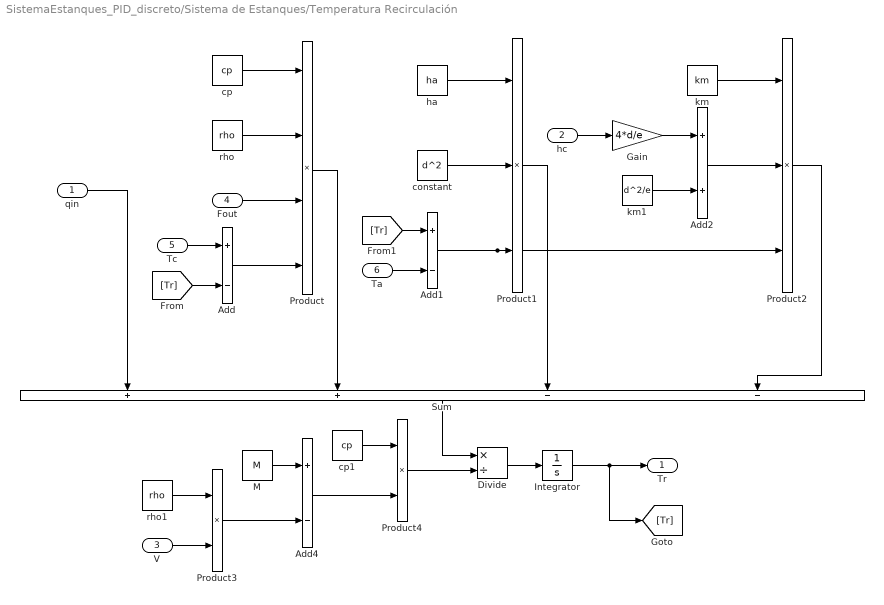
== system SistemaEstanques_PID_discreto/Sistema de Estanques/Temperatura Recirculación ==
  qin : Inport
  hc : Inport  Port=2
  V : Inport  Port=3
  Fout : Inport  Port=4
  Tc : Inport  Port=5
  Ta : Inport  Port=6
  Add : Sum  Inputs=+-
  Add1 : Sum  Inputs=+-
  Add2 : Sum
  Add4 : Sum  Inputs=+-
  Divide : Product  Inputs=*/
  Gain : Gain  Gain=4*d/e
  Integrator : Integrator  InitialCondition=T0r
  M : Constant  Value=M
  Product : Product  Inputs=4
  Product1 : Product  Inputs=3
  Product2 : Product  Inputs=3
  Product3 : Product
  Product4 : Product
  Sum : Sum  Inputs=++--
  constant : Constant  Value=d^2
  cp : Constant  Value=cp
  cp1 : Constant  Value=cp
  ha : Constant  Value=ha
  km : Constant  Value=km
  km1 : Constant  Value=d^2/e
  rho : Constant  Value=rho
  rho1 : Constant  Value=rho
  Tr : Outport
  wires:
  Integrator/1 -> Tr/1, [Tr]
  cp/1 -> Product/1
  rho/1 -> Product/2
  Fout/1 -> Product/3
  Add/1 -> Product/4
  Ta/1 -> Add1/2
  ha/1 -> Product1/1
  constant/1 -> Product1/2
  Add1/1 -> Product1/3, Product2/3
  hc/1 -> Gain/1
  Gain/1 -> Add2/1
  km1/1 -> Add2/2
  km/1 -> Product2/1
  Add2/1 -> Product2/2
  Product2/1 -> Sum/4
  Product1/1 -> Sum/3
  Product/1 -> Sum/2
  qin/1 -> Sum/1
  M/1 -> Add4/1
  Product3/1 -> Add4/2
  V/1 -> Product3/2
  rho1/1 -> Product3/1
  Add4/1 -> Product4/2
  cp1/1 -> Product4/1
  Product4/1 -> Divide/2
  Sum/1 -> Divide/1
  Divide/1 -> Integrator/1
  [Tr] -> Add/2
  Tc/1 -> Add/1
  [Tr] -> Add1/1
